simulink model "Integral_"  (R2020b)
settings: Solver=VariableStepAuto  StartTime=0.0  StopTime=10.0  RelTol=1e-3
settings Model: Creator=MSI  LastModifiedBy=MSI

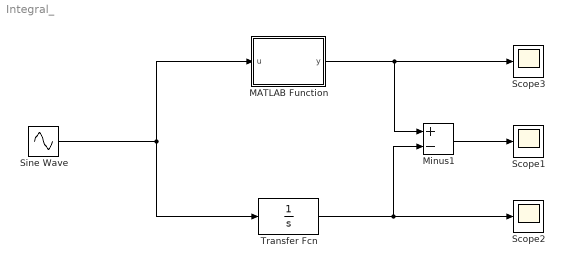
== system Integral_ ==
  MATLAB Function : MATLAB Function  TreatAsAtomicUnit=on
  Minus1 : Sum  Inputs=+-
  Scope1 : Scope
  Scope2 : Scope
  Scope3 : Scope
  Sine Wave : Sin  SampleTime=0
  Transfer Fcn : TransferFcn  Denominator=[1 0]
  wires:
  MATLAB Function/1(y) -> Minus1/1, Scope3/1
  Transfer Fcn/1 -> Minus1/2, Scope2/1
  Sine Wave/1 -> MATLAB Function/1(u), Transfer Fcn/1
  Minus1/1 -> Scope1/1

== matlab function Integral_/MATLAB Function ==
  settings: updateMethod=DISCRETE  sampleTime=1/500
  data: u input; y output
function y = Integral(u)

persistent Sum
Tsample = 1/500;

if isempty(Sum)
    Sum = 0;
end

Sum = Sum + u*Tsample;

y = Sum;
